simulink model "simple_ANSFT"  (R2023a)
settings: Solver=ode1  StartTime=0.0  StopTime=60  FixedStep=0.01  RelTol=1e-3
settings Model: Creator=Adan Daniel  LastModifiedBy=Adan Daniel
settings OptimizationCC: ReuseModelBlockBuffer=off

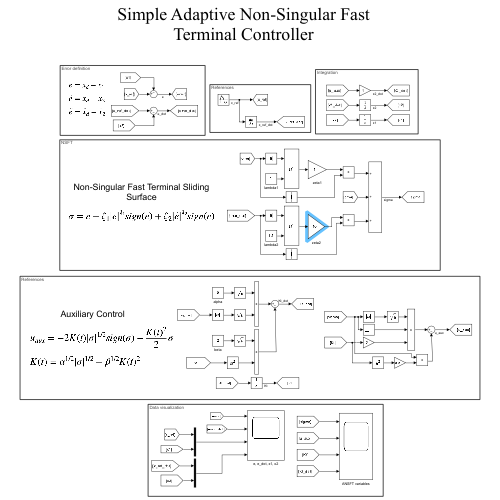
[thumbnail: Simulink's stored preview of the top-level diagram]
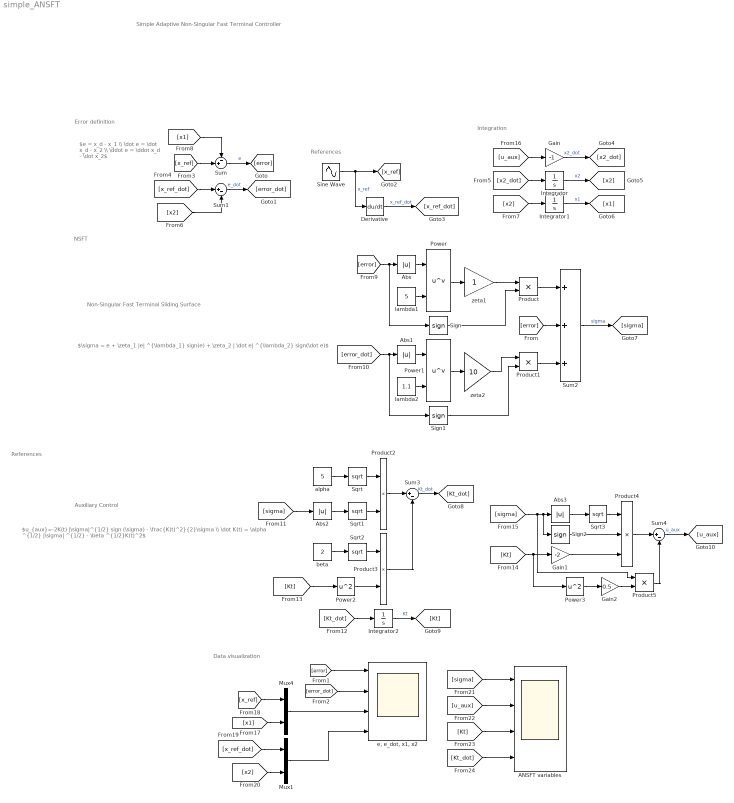
== system simple_ANSFT ==
  note: References
  note: Simple Adaptive Non-Singular Fast Terminal Controller
  note: $e = x_d - x_1 \\ \dot e = \dot x_d - x_2 \\ \ddot e = \ddot x_d - \dot x_2$
  note: Non-Singular Fast Terminal Sliding Surface
  note: $\sigma = e + \zeta_1 |e| ^{\lambda_1} sign(e) + \zeta_2 | \dot e| ^{\lambda_2} sign(\dot e)$
  note: Auxiliary Control
  note: $u_{aux}=-2K(t) |\sigma|^{1/2} sign (\sigma) - \frac{K(t)^2}{2}\sigma \\ \dot K(t) = \alpha ^{1/2} |\sigma| ^{1/2} - \beta ^{1/2}K(t)^2$
  note: Error definition
  note: NSFT
  note: References
  note: Integration
  note: Data visualization
  ANSFT variables : Scope  NumInputPorts=4
  Abs{,1..3} (4 alike) : Abs  SaturateOnIntegerOverflow=off
  Derivative : Derivative
  Gain : Gain  Gain=-1
  Gain1 : Gain  Gain=-2
  Gain2 : Gain  Gain=0.5
  Integrator : Integrator
  Integrator1 : Integrator
  Integrator2 : Integrator
  Mux1 : Mux  Inputs=2
  Mux4 : Mux  Inputs=2
  Power : Math  Operator=pow
  Power1 : Math  Operator=pow
  Power2 : Math  Operator=square
  Power3 : Math  Operator=square
  Product{,1..3,5} (5 alike) : Product
  Product4 : Product  Inputs=3
  Sign : Signum
  Sign1 : Signum
  Sign2 : Signum
  Sine Wave : Sin  Amplitude=0.8  Frequency=0.5  SampleTime=0
  Sqrt{,1..3} (4 alike) : Sqrt
  Sum : Sum  Inputs=-+|
  Sum1 : Sum  Inputs=|+-
  Sum2 : Sum  Inputs=+++
  Sum3 : Sum  Inputs=|+-
  Sum4 : Sum  Inputs=|+-
  alpha : Constant  Value=5
  beta : Constant  Value=2
  "e, e_dot, x1, x2" : Scope  NumInputPorts=4
  lambda1 : Constant  Value=5
  lambda2 : Constant  Value=1.1
  zeta1 : Gain
  zeta2 : Gain  Gain=10
  wires:
  Derivative/1 -> [x_ref_dot]  "x_ref_dot"
  Integrator1/1 -> [x1]  "x1"
  Integrator/1 -> [x2]  "x2"
  Sum/1 -> [error]  "e"
  Sum1/1 -> [error_dot]  "e_dot"
  Sum2/1 -> [sigma]  "sigma"
  Sum4/1 -> [u_aux]  "u_aux"
  Sum3/1 -> [Kt_dot]  "Kt_dot"
  Integrator2/1 -> [Kt]  "Kt"
  Sine Wave/1 -> [x_ref], Derivative/1  "x_ref"
  Abs/1 -> Power/1
  lambda1/1 -> Power/2
  Power/1 -> zeta1/1
  zeta1/1 -> Product/1
  Sign/1 -> Product/2
  Power1/1 -> zeta2/1
  Sign1/1 -> Product1/2
  lambda2/1 -> Power1/2
  zeta2/1 -> Product1/1
  Abs1/1 -> Power1/1
  Product1/1 -> Sum2/3
  alpha/1 -> Sqrt/1
  Abs2/1 -> Sqrt1/1
  Sqrt/1 -> Product2/1
  Sqrt1/1 -> Product2/2
  Product2/1 -> Sum3/1
  beta/1 -> Sqrt2/1
  Sqrt2/1 -> Product3/1
  Power2/1 -> Product3/2
  Product3/1 -> Sum3/2
  Abs3/1 -> Sqrt3/1
  Sqrt3/1 -> Product4/1
  Sign2/1 -> Product4/2
  Gain1/1 -> Product4/3
  Product4/1 -> Sum4/1
  Power3/1 -> Gain2/1
  Gain2/1 -> Product5/2
  Product5/1 -> Sum4/2
  [error] -> "e, e_dot, x1, x2"/1
  [x_ref] -> Sum/2
  [x_ref_dot] -> Sum1/1
  [x2_dot] -> Integrator/1
  [x2] -> Sum1/2
  [x2] -> Integrator1/1
  [x1] -> Sum/1
  [error] -> Sign/1, Abs/1
  [error_dot] -> Sign1/1, Abs1/1
  [error] -> Sum2/2
  Product/1 -> Sum2/1
  [sigma] -> Abs2/1
  [Kt_dot] -> Integrator2/1
  [Kt] -> Power2/1
  [sigma] -> Sign2/1, Abs3/1, Product5/1
  [Kt] -> Gain1/1, Power3/1
  Gain/1 -> [x2_dot]  "x2_dot"
  [u_aux] -> Gain/1
  [error_dot] -> "e, e_dot, x1, x2"/2
  [x1] -> Mux4/2
  [x_ref] -> Mux4/1
  [x_ref_dot] -> Mux1/1
  [x2] -> Mux1/2
  Mux4/1 -> "e, e_dot, x1, x2"/3
  Mux1/1 -> "e, e_dot, x1, x2"/4
  [Kt_dot] -> ANSFT variables/4
  [Kt] -> ANSFT variables/3
  [u_aux] -> ANSFT variables/2
  [sigma] -> ANSFT variables/1
